simulink model "lab_2_sqrt"  (R2012b)
settings: Solver=ode45  StartTime=0.0  StopTime=0.000036  FixedStep=Td  RelTol=1e-3
values from neighbouring files (symbols this model uses):
  Tb = 1/Rb    (= 1.11607142857e-06)    [lab_2_parameters.m]
undefined symbols (not defined in the file or in its folder): dfilt, rcosine
libraries: dspsigops x4, commsink2 x3, dsparch4 x2, dspmlti4 x2, commfilt2 x2, commrandsrc2 x1
settings Model: Creator=yuw  LastModifiedBy=yuw
settings OptimizationCC: InlineInvariantSignals=on  InitFltsAndDblsToZero=on
settings DebuggingCC: SaveWithParameterizedLinksMsg=none  SignalResolutionControl=TryResolveAllWithWarning  MultiTaskDSMMsg=warning  MultiTaskCondExecSysMsg=none  StrictBusMsg=None
settings RTWCC: IncludeERTFirstTime=on
settings GRTTargetCC: TargetFcnLib=ansi_tfl_tmw.mat  CombineOutputUpdateFcns=off  GRTInterface=on

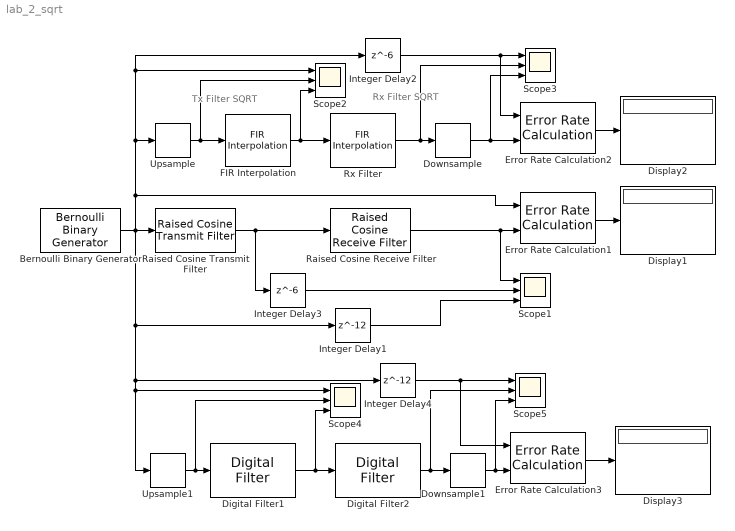
== system lab_2_sqrt ==
  note: Tx Filter SQRT
  note: Rx Filter SQRT
  Bernoulli Binary Generator : commrandsrc2/Bernoulli Binary Generator  P=0.5  seed=12345  Ts=Tb  frameBased=off  sampPerFrame=1  orient=off  outDataType=double
  Digital Filter1 : dsparch4/Digital Filter  TypePopup=FIR (all zeros)  IIRFiltStruct=Direct form II transposed  AllPoleFiltStruct=Direct form  FIRFiltStruct=Direct form  CoeffSource=Specify via dialog  NumCoeffs=[1 2]  DenCoeffs=[1 0.1]  BiQuadCoeffs=[1 0.3 0.4 1 0.1 0.2]  LatticeCoeffs=[0.2 0.4]  denIgnore=on  FiltPerSampPopup=One filter per frame  IC=0  ICnum=0  ICden=0  roundingMode=Floor  overflowMode=off  ScaleValues=1  scaleValueFracLength=14  stageInFracLength=15  stageOutFracLength=15  FilterSource=Specify via dialog  dfiltObjectName=dfilt.dffir([1 2 1])
  Digital Filter2 : dsparch4/Digital Filter  TypePopup=FIR (all zeros)  IIRFiltStruct=Direct form II transposed  AllPoleFiltStruct=Direct form  FIRFiltStruct=Direct form  CoeffSource=Specify via dialog  NumCoeffs=[1 2]  DenCoeffs=[1 0.1]  BiQuadCoeffs=[1 0.3 0.4 1 0.1 0.2]  LatticeCoeffs=[0.2 0.4]  denIgnore=on  FiltPerSampPopup=One filter per frame  IC=0  ICnum=0  ICden=0  roundingMode=Floor  overflowMode=off  ScaleValues=1  scaleValueFracLength=14  stageInFracLength=15  stageOutFracLength=15  FilterSource=Specify via dialog  dfiltObjectName=dfilt.dffir([1 2 1])
  Display1 : Display
  Display2 : Display
  Display3 : Display
  Downsample : dspsigops/Downsample  N=8  phase=0  RateOptions=Allow multirate processing  smode=Allow multirate  fmode=Maintain input frame size  ic=0
  Downsample1 : dspsigops/Downsample  N=8  phase=0  RateOptions=Allow multirate processing  smode=Allow multirate  fmode=Maintain input frame size  ic=0
  Error Rate Calculation1 : commsink2/Error Rate Calculation  N=0  st_delay=0  cp_mode=Entire frame  subframe=[]  PMode=Port  WsName=ErrorVec  RsMode2=off  stop=off  numErr=100  maxBits=1e6
  Error Rate Calculation2 : commsink2/Error Rate Calculation  N=0  st_delay=0  cp_mode=Entire frame  subframe=[]  PMode=Port  WsName=ErrorVec  RsMode2=off  stop=off  numErr=100  maxBits=1e6
  Error Rate Calculation3 : commsink2/Error Rate Calculation  N=0  st_delay=0  cp_mode=Entire frame  subframe=[]  PMode=Port  WsName=ErrorVec  RsMode2=off  stop=off  numErr=100  maxBits=1e6
  FIR Interpolation : dspmlti4/FIR Interpolation  h=rcosine(1, 8, 'sqrt', 0.5,3)  L=1  framing=Maintain input frame size  outputBufInitCond=0  firstCoeffDataTypeStr=Inherit: Same word length as input  firstCoeffLastDataTypeStr=Inherit: Same word length as input  firstCoeffMin=[]  firstCoeffMax=[]  outputDataTypeStr=Inherit: Same as accumulator  outputLastDataTypeStr=Inherit: Same as accumulator  outputMin=[]  outputMax=[]  roundingMode=Floor  overflowMode=off  FilterSource=Specify via dialog  FilterObject=Hm_firinterp
  Integer Delay1 : Delay  DelayLength=12  InputProcessing=Inherited
  Integer Delay2 : Delay  DelayLength=6  InputProcessing=Inherited
  Integer Delay3 : Delay  DelayLength=6  InputProcessing=Inherited
  Integer Delay4 : Delay  DelayLength=12  InputProcessing=Inherited
  Raised Cosine Receive Filter : commfilt2/Raised Cosine Receive Filter  filtType=Square root  N=8  D=6  R=0.2  sampMode=Mute  saveAsFlag=0  rateMode=Downsampling  downFactor=8  downOffset=0  framing=Maintain input frame size  checkGain=Normalized  filterGain=1  checkCoeff=on  variableName=rcRxFilt  launchFVT=off  roundingMode=Floor  overflowMode=off
  Raised Cosine Transmit Filter : commfilt2/Raised Cosine Transmit Filter  filtType=Square root  D=6  R=0.2  sampMode=Mute  saveAsFlag=0  N=8  framing=Maintain input frame size  checkGain=Normalized  filterGain=1  checkCoeff=on  variableName=rcTxFilt  launchFVT=off  roundingMode=Floor  overflowMode=off
  Rx Filter : dspmlti4/FIR Interpolation  h=rcosine(1, 8, 'sqrt', 0.5,3)  L=1  framing=Maintain input frame size  outputBufInitCond=0  firstCoeffDataTypeStr=Inherit: Same word length as input  firstCoeffLastDataTypeStr=Inherit: Same word length as input  firstCoeffMin=[]  firstCoeffMax=[]  outputDataTypeStr=Inherit: Same as accumulator  outputLastDataTypeStr=Inherit: Same as accumulator  outputMin=[]  outputMax=[]  roundingMode=Floor  overflowMode=off  FilterSource=Specify via dialog  FilterObject=Hm_firinterp
  Scope{1..5} (5 alike) : Scope  NumInputPorts=3
      Scope1 settings: TimeRange=5  YMin=-5~-5~-5  YMax=5~5~5  SaveName=ScopeData14
      Scope2 settings: TimeRange=5  YMin=-2~-2~-5  YMax=2~2~5  SaveName=ScopeData2
      Scope3 settings: TimeRange=5  YMin=-5~-5~-5  YMax=5~5~5  SaveName=ScopeData16
      Scope4 settings: TimeRange=5  YMin=-5~-5~-5  YMax=5~5~5  SaveName=ScopeData3
      Scope5 settings: TimeRange=5  YMin=-5~-5~-5  YMax=5~5~5  SaveName=ScopeData4
  Upsample : dspsigops/Upsample  N=8  phase=0  RateOptions=Allow multirate processing  ic=0  mode=Unused parameter value
  Upsample1 : dspsigops/Upsample  N=8  phase=0  RateOptions=Allow multirate processing  ic=0  mode=Unused parameter value
  wires:
  Raised Cosine Transmit Filter/1 -> Integer Delay3/1, Raised Cosine Receive Filter/1
  Bernoulli Binary Generator/1 -> Raised Cosine Transmit Filter/1, Integer Delay1/1, Upsample1/1, Scope4/1, Integer Delay4/1, Upsample/1, Scope2/1, Integer Delay2/1, Error Rate Calculation1/1
  Error Rate Calculation1/1 -> Display1/1
  Raised Cosine Receive Filter/1 -> Error Rate Calculation1/2, Scope1/1
  Error Rate Calculation2/1 -> Display2/1
  Downsample/1 -> Error Rate Calculation2/2, Scope3/3
  Upsample/1 -> Scope2/2, FIR Interpolation/1
  Integer Delay2/1 -> Scope3/1, Error Rate Calculation2/1
  Upsample1/1 -> Digital Filter1/1, Scope4/2
  Digital Filter1/1 -> Digital Filter2/1, Scope4/3
  Digital Filter2/1 -> Downsample1/1, Scope5/2
  Error Rate Calculation3/1 -> Display3/1
  Downsample1/1 -> Error Rate Calculation3/2, Scope5/3
  Integer Delay4/1 -> Scope5/1, Error Rate Calculation3/1
  Integer Delay3/1 -> Scope1/2
  Integer Delay1/1 -> Scope1/3
  FIR Interpolation/1 -> Scope2/3, Rx Filter/1
  Rx Filter/1 -> Scope3/2, Downsample/1
